simulink model "RRmanipulatorsim"  (R2020a)
settings: Solver=VariableStepAuto  StartTime=0.0  StopTime=7  RelTol=1e-3
values from neighbouring files (symbols this model uses):
  ike = ke^(-1)    (= 1e-06)    [RRmanipulator.m]    (also in RRmanipulator_.m)
  Ke = [1e6 0; 0 0]    [RRmanipulator.m]    (also in RRmanipulator_.m)
  ke = 1e6    (= 1000000)    [RRmanipulator.m]    (also in RRmanipulator_.m)
  Kp = [g1 0; 0 g2]    [RRmanipulator.m]    (also in RRmanipulator_.m)
  Kpf = [g1f 0; 0 g2f]    [RRmanipulator.m]    (also in RRmanipulator_.m)
  Kpf_ = g1f    (= 500000)    [RRmanipulator.m]    (also in RRmanipulator_.m)
  Kv = [2*sqrt(g1) 0; 0 2*sqrt(g2)]    [RRmanipulator.m]    (also in RRmanipulator_.m)
  Kvf = [2*sqrt(g1f) 0; 0 2*sqrt(g2f)]    [RRmanipulator.m]    (also in RRmanipulator_.m)
  R = [cos(-pi/4) -sin(-pi/4) ... (first row only)    [RRmanipulator.m]    (also in RRmanipulator_.m)
  RT = R'    [RRmanipulator.m]    (also in RRmanipulator_.m)
  S = [0 0; 0 1]    [RRmanipulator.m]    (also in RRmanipulator_.m)
  S_ = [1 0; 0 0]    [RRmanipulator.m]    (also in RRmanipulator_.m)
libraries: roblocks x29, simulink x11
(part 1 of 2)
settings Model: Creator=Tobias Scala  LastModifiedBy=Tobias Scala

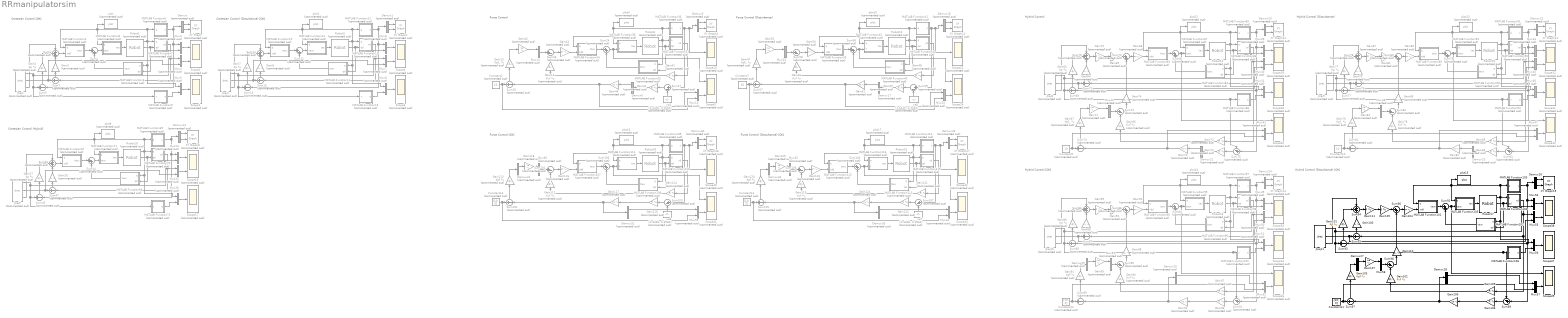
== system RRmanipulatorsim ==
  note: Cartesian Control [OK]
  note: Cartesian Control (Disturbance) [OK]
  note: Force Control
  note: Cartesian Control (Hybrid)
  note: Force Control (Disturbance)
  note: Hybrid Control
  note: Hybrid Control (Disturbance)
  note: Hybrid Control (Disturbance) [OK]
  note: Hybrid Control [OK]
  note: Force Control [OK]
  note: Force Control (Disturbance) [OK]
  Constant{2,7,9..10} (4 alike) : Constant  Commented=on  Value=10
  Constant11 : Constant  Value=[10; 0]
  Constant12 : Constant  Commented=on  Value=[10; 0]
  Constant13 : Constant  Commented=on  Value=[10; 0]
  Constant14 : Constant  Commented=on  Value=[10; 0]
  Demux{,1,5..6,13,16..17,20..25,29..35} (20 alike) : Demux  Commented=on  Outputs=2
  Demux26 : Demux  Outputs=2
  Demux27 : Demux  Outputs=2
  Demux28 : Demux  Outputs=2
  Gain100 : Gain  Gain=Kv  Multiplication=Matrix(K*u)
  Gain101 : Gain  Gain=Kp  Multiplication=Matrix(K*u)
  Gain102 : Gain  Gain=Kvf  Multiplication=Matrix(K*u)
  Gain103 : Gain  Gain=Kpf  Multiplication=Matrix(K*u)
  Gain104 : Gain  Gain=RT  Multiplication=Matrix(K*u)
  Gain105 : Gain  Gain=S  Multiplication=Matrix(K*u)
  Gain106 : Gain  Gain=Ke  Multiplication=Matrix(K*u)
  Gain107 : Gain  Gain=ike  Multiplication=Matrix(K*u)
  Gain108 : Gain  Gain=R  Multiplication=Matrix(K*u)
  Gain109 : Gain  Gain=R  Multiplication=Matrix(K*u)
  Gain110 : Gain  Gain=S_  Multiplication=Matrix(K*u)
  Gain111 : Gain  Gain=R  Multiplication=Matrix(K*u)
  Gain{12,46,66,78,90,112,119} (7 alike) : Gain  Commented=on  Gain=Kvf  Multiplication=Matrix(K*u)
  Gain113 : Gain  Commented=on  Gain=Kpf  Multiplication=Matrix(K*u)
  Gain{41..42,48..49,72..73,75,84..85,87,96..97,99,114..115,121..122} (17 alike) : Gain  Commented=on  Gain=R  Multiplication=Matrix(K*u)
  Gain{43,50,68,80,92,116,123} (7 alike) : Gain  Commented=on  Gain=RT  Multiplication=Matrix(K*u)
  Gain117 : Gain  Commented=on  Gain=Ke  Multiplication=Matrix(K*u)
  Gain{45,52,71,83,95,118,125} (7 alike) : Gain  Commented=on  Gain=ike  Multiplication=Matrix(K*u)
  Gain120 : Gain  Commented=on  Gain=Kpf  Multiplication=Matrix(K*u)
  Gain124 : Gain  Commented=on  Gain=Ke  Multiplication=Matrix(K*u)
  Gain{13,47,67,79} (4 alike) : Gain  Commented=on  Gain=Kpf_  Multiplication=Matrix(K*u)
  Gain{2,6,26,64,76,88} (6 alike) : Gain  Commented=on  Gain=Kv  Multiplication=Matrix(K*u)
  Gain{3,7,27,65,77,89} (6 alike) : Gain  Commented=on  Gain=Kp  Multiplication=Matrix(K*u)
  Gain{44,51,70,82} (4 alike) : Gain  Commented=on  Gain=ke  Multiplication=Matrix(K*u)
  Gain69 : Gain  Commented=on  Gain=S  Multiplication=Matrix(K*u)
  Gain74 : Gain  Commented=on  Gain=S_  Multiplication=Matrix(K*u)
  Gain81 : Gain  Commented=on  Gain=S  Multiplication=Matrix(K*u)
  Gain86 : Gain  Commented=on  Gain=S_  Multiplication=Matrix(K*u)
  Gain91 : Gain  Commented=on  Gain=Kpf  Multiplication=Matrix(K*u)
  Gain93 : Gain  Commented=on  Gain=S  Multiplication=Matrix(K*u)
  Gain94 : Gain  Commented=on  Gain=Ke  Multiplication=Matrix(K*u)
  Gain98 : Gain  Commented=on  Gain=S_  Multiplication=Matrix(K*u)
  MATLAB Function10 : MATLAB Function  Commented=on  TreatAsAtomicUnit=on
  MATLAB Function100 : MATLAB Function  Commented=on  TreatAsAtomicUnit=on
  MATLAB Function101 : MATLAB Function  TreatAsAtomicUnit=on
  MATLAB Function102 : MATLAB Function  TreatAsAtomicUnit=on
  MATLAB Function103 : MATLAB Function  TreatAsAtomicUnit=on
  MATLAB Function104 : MATLAB Function  TreatAsAtomicUnit=on
  MATLAB Function105 : MATLAB Function  TreatAsAtomicUnit=on
  MATLAB Function106 : MATLAB Function  TreatAsAtomicUnit=on
  MATLAB Function107 : MATLAB Function  Commented=on  TreatAsAtomicUnit=on
  MATLAB Function108 : MATLAB Function  Commented=on  TreatAsAtomicUnit=on
  MATLAB Function109 : MATLAB Function  Commented=on  TreatAsAtomicUnit=on
  MATLAB Function11 : MATLAB Function  Commented=on  TreatAsAtomicUnit=on
  MATLAB Function110 : MATLAB Function  Commented=on  TreatAsAtomicUnit=on
  MATLAB Function111 : MATLAB Function  Commented=on  TreatAsAtomicUnit=on
  MATLAB Function112 : MATLAB Function  Commented=on  TreatAsAtomicUnit=on
  MATLAB Function113 : MATLAB Function  Commented=on  TreatAsAtomicUnit=on
  MATLAB Function114 : MATLAB Function  Commented=on  TreatAsAtomicUnit=on
  MATLAB Function115 : MATLAB Function  Commented=on  TreatAsAtomicUnit=on
  MATLAB Function116 : MATLAB Function  Commented=on  TreatAsAtomicUnit=on
  MATLAB Function12 : MATLAB Function  Commented=on  TreatAsAtomicUnit=on
  MATLAB Function13 : MATLAB Function  Commented=on  TreatAsAtomicUnit=on
  MATLAB Function14 : MATLAB Function  Commented=on  TreatAsAtomicUnit=on
  MATLAB Function15 : MATLAB Function  Commented=on  TreatAsAtomicUnit=on
  MATLAB Function2 : MATLAB Function  Commented=on  TreatAsAtomicUnit=on
  MATLAB Function3 : MATLAB Function  Commented=on  TreatAsAtomicUnit=on
  MATLAB Function34 : MATLAB Function  Commented=on  TreatAsAtomicUnit=on
  MATLAB Function35 : MATLAB Function  Commented=on  TreatAsAtomicUnit=on
  MATLAB Function36 : MATLAB Function  Commented=on  TreatAsAtomicUnit=on
  MATLAB Function37 : MATLAB Function  Commented=on  TreatAsAtomicUnit=on
  MATLAB Function38 : MATLAB Function  Commented=on  TreatAsAtomicUnit=on
  MATLAB Function39 : MATLAB Function  Commented=on  TreatAsAtomicUnit=on
  MATLAB Function40 : MATLAB Function  Commented=on  TreatAsAtomicUnit=on
  MATLAB Function41 : MATLAB Function  Commented=on  TreatAsAtomicUnit=on
  MATLAB Function42 : MATLAB Function  Commented=on  TreatAsAtomicUnit=on
  MATLAB Function43 : MATLAB Function  Commented=on  TreatAsAtomicUnit=on
  MATLAB Function6 : MATLAB Function  Commented=on  TreatAsAtomicUnit=on
  MATLAB Function67 : MATLAB Function  Commented=on  TreatAsAtomicUnit=on
  MATLAB Function68 : MATLAB Function  Commented=on  TreatAsAtomicUnit=on
  MATLAB Function69 : MATLAB Function  Commented=on  TreatAsAtomicUnit=on
  MATLAB Function7 : MATLAB Function  Commented=on  TreatAsAtomicUnit=on
  MATLAB Function70 : MATLAB Function  Commented=on  TreatAsAtomicUnit=on
  MATLAB Function71 : MATLAB Function  Commented=on  TreatAsAtomicUnit=on
  MATLAB Function72 : MATLAB Function  Commented=on  TreatAsAtomicUnit=on
  MATLAB Function8 : MATLAB Function  Commented=on  TreatAsAtomicUnit=on
  MATLAB Function83 : MATLAB Function  Commented=on  TreatAsAtomicUnit=on
  MATLAB Function84 : MATLAB Function  Commented=on  TreatAsAtomicUnit=on
  MATLAB Function85 : MATLAB Function  Commented=on  TreatAsAtomicUnit=on
  MATLAB Function86 : MATLAB Function  Commented=on  TreatAsAtomicUnit=on
  MATLAB Function87 : MATLAB Function  Commented=on  TreatAsAtomicUnit=on
  MATLAB Function88 : MATLAB Function  Commented=on  TreatAsAtomicUnit=on
  MATLAB Function89 : MATLAB Function  Commented=on  TreatAsAtomicUnit=on
  MATLAB Function9 : MATLAB Function  Commented=on  TreatAsAtomicUnit=on
  MATLAB Function90 : MATLAB Function  Commented=on  TreatAsAtomicUnit=on
  MATLAB Function91 : MATLAB Function  Commented=on  TreatAsAtomicUnit=on
  MATLAB Function92 : MATLAB Function  Commented=on  TreatAsAtomicUnit=on
  MATLAB Function93 : MATLAB Function  Commented=on  TreatAsAtomicUnit=on
  MATLAB Function94 : MATLAB Function  Commented=on  TreatAsAtomicUnit=on
  MATLAB Function95 : MATLAB Function  Commented=on  TreatAsAtomicUnit=on
  MATLAB Function96 : MATLAB Function  Commented=on  TreatAsAtomicUnit=on
  MATLAB Function97 : MATLAB Function  Commented=on  TreatAsAtomicUnit=on
  MATLAB Function98 : MATLAB Function  Commented=on  TreatAsAtomicUnit=on
  MATLAB Function99 : MATLAB Function  Commented=on  TreatAsAtomicUnit=on
  Mux{3..8,13..14,24..26,32..33,39..53,59..62} (32 alike) : Mux  Commented=on  Inputs=2
  Mux{54..58} (5 alike) : Mux  Inputs=2
  Robot1 : roblocks/Arm/Robot  Commented=on  robot=RRbot  q0=[-pi/2 pi/2]
  Robot{6,10,14,16,18} (5 alike) : roblocks/Arm/Robot  Commented=on  robot=RRbot  q0=[-0.114*pi 0.364*pi]
  Robot12 : roblocks/Arm/Robot  Commented=on  robot=RRbotD  q0=[-0.114*pi 0.364*pi]
  Robot15 : roblocks/Arm/Robot  Commented=on  robot=RRbotD  q0=[-0.114*pi 0.364*pi]
  Robot17 : roblocks/Arm/Robot  robot=RRbotD  q0=[-0.114*pi 0.364*pi]
  Robot19 : roblocks/Arm/Robot  Commented=on  robot=RRbotD  q0=[-0.114*pi 0.364*pi]
  Robot3 : roblocks/Arm/Robot  Commented=on  robot=RRbotD  q0=[-pi/2 pi/2]
  Scope{1,3,10,17,23,28,31,34,40,42} (10 alike) : Scope  Commented=on
  Scope{2,4,9,19,24,29..30,32..33,35..36,41,43} (13 alike) : Scope  Commented=on  NumInputPorts=2
  Scope37 : Scope
  Scope38 : Scope  NumInputPorts=2
  Scope39 : Scope  NumInputPorts=2
  Sum{4,12,24,44,56,68,72,76,80,84,88,100,104} (13 alike) : Sum  Commented=on  Inputs=|++
  Sum{5,7,13,15,25,45,47,57,69,71,73,77,79,81,85,87,89,101,105} (19 alike) : Sum  Commented=on  Inputs=+|-
  Sum{26..27,58..59,74,82,90,102..103,106..107} (11 alike) : Sum  Commented=on  Inputs=|+-
  Sum{6,14,46,70,78,86} (6 alike) : Sum  Commented=on  Inputs=+++
  Sum75 : Sum  Commented=on  Inputs=-+|
  Sum83 : Sum  Commented=on  Inputs=-+|
  Sum91 : Sum  Commented=on  Inputs=-+|
  Sum92 : Sum  Inputs=|++
  Sum93 : Sum  Inputs=+|-
  Sum94 : Sum  Inputs=+++
  Sum95 : Sum  Inputs=+|-
  Sum96 : Sum  Inputs=|++
  Sum97 : Sum  Inputs=+|-
  Sum98 : Sum  Inputs=|+-
  Sum99 : Sum  Inputs=-+|
  XY Graph{,1,4,10,16..17} (6 alike) : simulink/Sinks/XY Graph  Commented=on  xmin=-1.5  xmax=1.5  ymin=-1.5  ymax=1.5  st=-1
  XY Graph{8,12..14} (4 alike) : simulink/Sinks/XY Graph  Commented=on  xmin=-2  xmax=2  ymin=-2  ymax=2  st=-1
  XY Graph15 : simulink/Sinks/XY Graph  xmin=-2  xmax=2  ymin=-2  ymax=2  st=-1
  jtraj1 : roblocks/Toolbox/jtraj  Commented=on  q0=[1 -1]  qf=[1 1]  tmax=2  ts=0.02
  jtraj{5,8..10} (4 alike) : roblocks/Toolbox/jtraj  Commented=on  q0=[1.6436 0.3564]  qf=[0.3564 1.6436]  tmax=2  ts=0.02
  jtraj11 : roblocks/Toolbox/jtraj  q0=[1.6436 0.3564]  qf=[0.3564 1.6436]  tmax=2  ts=0.02
  jtraj3 : roblocks/Toolbox/jtraj  Commented=on  q0=[1 -1]  qf=[1 1]  tmax=2  ts=0.02
  plot{,4,8,12,14,16} (6 alike) : roblocks/Arm/plot  Commented=on  robot=RRbot  fps=5  holdplot=on
  plot{1,10,13,17} (4 alike) : roblocks/Arm/plot  Commented=on  robot=RRbotD  fps=5  holdplot=on
  plot15 : roblocks/Arm/plot  robot=RRbotD  fps=5  holdplot=on
  xe{2,5..7} (4 alike) : Constant  Commented=on  Value=[1.6436; 0.3564]
  wires:
  jtraj1/3 -> Sum6/1
  jtraj1/1 -> MATLAB Function9/1(x), Sum5/1, Mux3/2
  Gain3/1 -> Sum6/2
  Sum7/1 -> Gain2/1
  jtraj1/2 -> Mux4/2, Sum7/1
  Sum5/1 -> Gain3/1
  Gain2/1 -> Sum6/3
  MATLAB Function3/1(taux) -> Sum4/2
  Robot1/1 -> MATLAB Function6/1(q), plot/1, MATLAB Function8/1(q), MATLAB Function2/1(q), Mux5/1, MATLAB Function3/1(q), MATLAB Function7/1(q)
  Robot1/2 -> MATLAB Function3/2(qd), MATLAB Function7/2(qd)
  Sum6/1 -> MATLAB Function2/2(xdd)
  MATLAB Function6/1(x) -> Demux/1, Sum5/2, Mux3/1
  MATLAB Function7/1(xd) -> Sum7/2, Mux4/1
  MATLAB Function2/1(taux) -> Sum4/1
  Sum4/1 -> MATLAB Function8/2(taux)
  MATLAB Function8/1(tau) -> Robot1/1
  Mux3/1 -> Scope2/1
  Mux4/1 -> Scope2/2
  Mux5/1 -> Scope1/1
  MATLAB Function9/1(q) -> Mux5/2
  Demux/2 -> XY Graph/2
  Demux/1 -> XY Graph/1
  MATLAB Function15/1(q) -> Mux8/2
  Demux1/2 -> XY Graph1/2
  MATLAB Function10/1(taux) -> Sum12/1
  Mux6/1 -> Scope4/1
  MATLAB Function14/1(tau) -> Robot3/1
  Mux8/1 -> Scope3/1
  Mux7/1 -> Scope4/2
  MATLAB Function12/1(x) -> Demux1/1, Sum13/2, Mux6/1
  Demux1/1 -> XY Graph1/1
  Robot3/2 -> MATLAB Function11/2(qd), MATLAB Function13/2(qd)
  Sum12/1 -> MATLAB Function14/2(taux)
  MATLAB Function13/1(xd) -> Sum15/2, Mux7/1
  Robot3/1 -> MATLAB Function12/1(q), plot1/1, MATLAB Function14/1(q), MATLAB Function10/1(q), Mux8/1, MATLAB Function11/1(q), MATLAB Function13/1(q)
  Sum14/1 -> MATLAB Function10/2(xdd)
  Sum13/1 -> Gain7/1
  Gain6/1 -> Sum14/3
  Gain7/1 -> Sum14/2
  jtraj3/3 -> Sum14/1
  jtraj3/2 -> Mux7/2, Sum15/1
  Sum15/1 -> Gain6/1
  jtraj3/1 -> MATLAB Function15/1(x), Sum13/1, Mux6/2
  MATLAB Function11/1(taux) -> Sum12/2
  MATLAB Function36/1(x) -> Demux5/1, Scope10/1, Sum27/1
  Constant2/1 -> Mux13/2, Sum25/1
  xe2/1 -> Sum27/2
  Sum27/1 -> Gain42/1
  Sum26/1 -> Gain43/1
  Gain44/1 -> Mux13/1, Sum25/2
  Gain45/1 -> Mux14/1
  Robot6/2 -> MATLAB Function35/2(qd), MATLAB Function37/2(qd)
  Sum24/1 -> Scope9/1, MATLAB Function38/2(f)
  Sum25/1 -> Gain13/1
  MATLAB Function34/1(taux) -> Sum24/1
  MATLAB Function35/1(taux) -> Sum24/2
  Demux6/1 -> Gain44/1
  MATLAB Function38/1(tau) -> Robot6/1
  Gain41/1 -> Gain12/1
  Demux5/1 -> XY Graph4/1
  Demux5/2 -> XY Graph4/2
  Gain43/1 -> MATLAB Function34/2(xdd)
  Gain12/1 -> Sum26/2
  MATLAB Function37/1(xd) -> Gain41/1
  Mux14/1 -> Sum26/1
  Robot6/1 -> MATLAB Function36/1(q), MATLAB Function38/1(q), MATLAB Function34/1(q), plot4/1, MATLAB Function35/1(q), MATLAB Function37/1(q)
  Gain42/1 -> Demux6/1
  Gain13/1 -> Gain45/1
  Mux13/1 -> Scope9/2
  Robot10/2 -> MATLAB Function68/2(qd), MATLAB Function70/2(qd)
  MATLAB Function67/1(taux) -> Sum44/1
  Sum44/1 -> MATLAB Function71/2(taux)
  Mux25/1 -> Scope19/2
  Sum46/1 -> MATLAB Function67/2(xdd)
  Gain27/1 -> Sum46/2
  Sum45/1 -> Gain27/1
  MATLAB Function70/1(xd) -> Sum47/2, Mux25/1
  MATLAB Function71/1(tau) -> Robot10/1
  MATLAB Function69/1(x) -> Demux13/1, Sum45/2, Mux24/1
  Robot10/1 -> MATLAB Function69/1(q), plot8/1, MATLAB Function71/1(q), MATLAB Function67/1(q), Mux26/1, MATLAB Function68/1(q), MATLAB Function70/1(q)
  Mux24/1 -> Scope19/1
  Mux26/1 -> Scope17/1
  Gain26/1 -> Sum46/3
  jtraj5/2 -> Mux25/2, Sum47/1
  Demux13/2 -> XY Graph8/2
  Sum47/1 -> Gain26/1
  MATLAB Function68/1(taux) -> Sum44/2
  Demux13/1 -> XY Graph8/1
  jtraj5/1 -> MATLAB Function72/1(x), Sum45/1, Mux24/2
  MATLAB Function72/1(q) -> Mux26/2
  jtraj5/3 -> Sum46/1
  Gain51/1 -> Mux32/1, Sum57/2
  Demux17/1 -> Gain51/1
  Gain49/1 -> Demux17/1
  MATLAB Function42/1(xd) -> Gain48/1
  Gain52/1 -> Mux33/1
  Gain47/1 -> Gain52/1
  Demux16/2 -> XY Graph10/2
  Sum56/1 -> Scope24/1, MATLAB Function43/2(f)
  Sum58/1 -> Gain50/1
  Mux33/1 -> Sum58/1
  Gain48/1 -> Gain46/1
  Mux32/1 -> Scope24/2
  Robot12/1 -> MATLAB Function41/1(q), MATLAB Function43/1(q), MATLAB Function39/1(q), plot10/1, MATLAB Function40/1(q), MATLAB Function42/1(q)
  Gain46/1 -> Sum58/2
  Demux16/1 -> XY Graph10/1
  MATLAB Function43/1(tau) -> Robot12/1
  Constant7/1 -> Mux32/2, Sum57/1
  MATLAB Function39/1(taux) -> Sum56/1
  xe5/1 -> Sum59/2
  Sum59/1 -> Gain49/1
  MATLAB Function41/1(x) -> Demux16/1, Scope23/1, Sum59/1
  Robot12/2 -> MATLAB Function40/2(qd), MATLAB Function42/2(qd)
  Gain50/1 -> MATLAB Function39/2(xdd)
  Sum57/1 -> Gain47/1
  MATLAB Function40/1(taux) -> Sum56/2
  Gain73/1 -> Gain66/1
  Gain66/1 -> Sum74/2
  MATLAB Function88/1(q) -> Mux41/2
  MATLAB Function87/1(tau) -> Robot14/1
  Demux21/1 -> Gain70/1
  MATLAB Function84/1(taux) -> Sum68/2
  Mux43/1 -> Sum74/1
  Gain70/1 -> Mux42/1, Sum73/2
  Sum75/1 -> Gain72/1
  Mux42/1 -> Scope30/2
  Sum71/1 -> Gain64/1
  Gain65/1 -> Sum70/2
  Robot14/1 -> MATLAB Function85/1(q), plot12/1, MATLAB Function87/1(q), MATLAB Function83/1(q), Mux41/1, MATLAB Function84/1(q), MATLAB Function86/1(q)
  Gain72/1 -> Demux21/1
  MATLAB Function85/1(x) -> Sum75/2, Sum69/2, Mux39/1, Demux20/1
  Constant9/1 -> Mux42/2, Sum73/1
  Demux20/2 -> XY Graph12/2
  Mux41/1 -> Scope28/1
  Gain64/1 -> Sum70/3
  Gain71/1 -> Mux43/1
  Sum68/1 -> Scope30/1, MATLAB Function87/2(taux)
  MATLAB Function83/1(taux) -> Sum68/1
  Sum74/1 -> Gain74/1
  Gain74/1 -> Sum72/2
  Sum69/1 -> Gain65/1
  Sum73/1 -> Gain67/1
  Gain69/1 -> Sum72/1
  MATLAB Function86/1(xd) -> Sum71/2, Gain73/1, Mux40/1
  Gain67/1 -> Gain71/1
  Demux20/1 -> XY Graph12/1
  Sum72/1 -> Gain68/1
  Sum70/1 -> Gain75/1
  Mux40/1 -> Scope29/2
  Robot14/2 -> MATLAB Function84/2(qd), MATLAB Function86/2(qd)
  Mux39/1 -> Scope29/1
  jtraj8/1 -> Mux39/2, Sum69/1, MATLAB Function88/1(x), Sum75/1
  jtraj8/2 -> Mux40/2, Sum71/1
  jtraj8/3 -> Sum70/1
  Gain68/1 -> MATLAB Function83/2(xdd)
  Gain75/1 -> Gain69/1
  Gain87/1 -> Gain81/1
  Mux45/1 -> Scope32/2
  Sum78/1 -> Gain87/1
  Sum80/1 -> Gain80/1
  Demux22/1 -> XY Graph13/1
  Gain79/1 -> Gain83/1
  MATLAB Function92/1(xd) -> Sum79/2, Gain85/1, Mux45/1
  MATLAB Function89/1(taux) -> Sum76/1
  Gain83/1 -> Mux48/1
  Sum76/1 -> Scope33/1, MATLAB Function93/2(taux)
  Demux22/2 -> XY Graph13/2
  Constant10/1 -> Mux47/2, Sum81/1
  Gain76/1 -> Sum78/3
  Sum82/1 -> Gain86/1
  Sum81/1 -> Gain79/1
  Gain77/1 -> Sum78/2
  Sum79/1 -> Gain76/1
  Mux47/1 -> Scope33/2
  Gain82/1 -> Mux47/1, Sum81/2
  Gain84/1 -> Demux23/1
  Gain81/1 -> Sum80/1
  MATLAB Function90/1(taux) -> Sum76/2
  Robot15/1 -> MATLAB Function91/1(q), plot13/1, MATLAB Function93/1(q), MATLAB Function89/1(q), Mux46/1, MATLAB Function90/1(q), MATLAB Function92/1(q)
  Sum77/1 -> Gain77/1
  Sum83/1 -> Gain84/1
  MATLAB Function93/1(tau) -> Robot15/1
  Demux23/1 -> Gain82/1
  Gain78/1 -> Sum82/2
  Gain85/1 -> Gain78/1
  MATLAB Function94/1(q) -> Mux46/2
  Robot15/2 -> MATLAB Function90/2(qd), MATLAB Function92/2(qd)
  jtraj9/2 -> Mux45/2, Sum79/1
  Mux48/1 -> Sum82/1
  jtraj9/1 -> Mux44/2, Sum77/1, MATLAB Function94/1(x), Sum83/1
  Mux46/1 -> Scope31/1
  jtraj9/3 -> Sum78/1
  Gain86/1 -> Sum80/2
  Mux44/1 -> Scope32/1
  Gain80/1 -> MATLAB Function89/2(xdd)
  MATLAB Function91/1(x) -> Sum83/2, Sum77/2, Mux44/1, Demux22/1
  Gain105/1 -> Sum96/1
  MATLAB Function102/1(taux) -> Sum92/2
  Sum98/1 -> Gain110/1
  Gain101/1 -> Sum94/2
  Sum97/1 -> Gain103/1
  Gain106/1 -> Demux28/1, Sum97/2
  Mux57/1 -> Scope39/2
  Sum95/1 -> Gain100/1
  Gain100/1 -> Sum94/3
  Demux26/2 -> XY Graph15/2
  Sum92/1 -> Scope39/1, MATLAB Function105/2(taux)
  MATLAB Function104/1(xd) -> Sum95/2, Gain109/1, Mux55/1
  MATLAB Function101/1(taux) -> Sum92/1
  Gain107/1 -> Mux58/1
  Sum99/1 -> Gain108/1
  Sum93/1 -> Gain101/1
  Robot17/1 -> MATLAB Function103/1(q), plot15/1, MATLAB Function105/1(q), MATLAB Function101/1(q), Mux56/1, MATLAB Function102/1(q), MATLAB Function104/1(q)
  Mux55/1 -> Scope38/2
  Constant11/1 -> Mux57/2, Sum97/1
  Sum94/1 -> Gain111/1
  Gain109/1 -> Gain102/1
  Gain102/1 -> Sum98/2
  jtraj11/2 -> Mux55/2, Sum95/1
  Robot17/2 -> MATLAB Function102/2(qd), MATLAB Function104/2(qd)
  Gain111/1 -> Gain105/1
  Gain110/1 -> Sum96/2
  Mux56/1 -> Scope37/1
  jtraj11/3 -> Sum94/1
  jtraj11/1 -> Mux54/2, Sum93/1, MATLAB Function106/1(x), Sum99/1
  Gain104/1 -> MATLAB Function101/2(xdd)
  MATLAB Function106/1(q) -> Mux56/2
  Mux58/1 -> Sum98/1
  MATLAB Function103/1(x) -> Sum99/2, Sum93/2, Mux54/1, Demux26/1
  Demux26/1 -> XY Graph15/1
  Sum96/1 -> Gain104/1
  Gain108/1 -> Gain106/1
  MATLAB Function105/1(tau) -> Robot17/1
  Mux54/1 -> Scope38/1
  Demux27/1 -> Gain107/1
  Gain103/1 -> Demux27/1
  Demux28/1 -> Mux57/1
  Mux49/1 -> Scope35/1
  Sum88/1 -> Gain92/1
  Demux24/1 -> XY Graph14/1
  MATLAB Function97/1(x) -> Sum91/2, Sum85/2, Mux49/1, Demux24/1
  Mux53/1 -> Sum90/1
  jtraj10/1 -> Mux49/2, Sum85/1, MATLAB Function100/1(x), Sum91/1
  Gain96/1 -> Gain94/1
  Gain99/1 -> Gain93/1
  Gain90/1 -> Sum90/2
  Gain97/1 -> Gain90/1
  MATLAB Function100/1(q) -> Mux51/2
  Mux50/1 -> Scope35/2
  Robot16/1 -> MATLAB Function97/1(q), plot14/1, MATLAB Function99/1(q), MATLAB Function95/1(q), Mux51/1, MATLAB Function96/1(q), MATLAB Function98/1(q)
  Gain92/1 -> MATLAB Function95/2(xdd)
  Sum85/1 -> Gain89/1
  jtraj10/2 -> Mux50/2, Sum87/1
  Robot16/2 -> MATLAB Function96/2(qd), MATLAB Function98/2(qd)
  Sum91/1 -> Gain96/1
  Gain95/1 -> Mux53/1
  jtraj10/3 -> Sum86/1
  Gain98/1 -> Sum88/2
  Constant12/1 -> Mux52/2, Sum89/1
  Mux51/1 -> Scope34/1
  Gain91/1 -> Demux25/1
  Demux29/1 -> Mux52/1
  MATLAB Function95/1(taux) -> Sum84/1
  Sum86/1 -> Gain99/1
  MATLAB Function99/1(tau) -> Robot16/1
  Sum84/1 -> Scope36/1, MATLAB Function99/2(taux)
  Demux24/2 -> XY Graph14/2
  Gain88/1 -> Sum86/3
  MATLAB Function98/1(xd) -> Sum87/2, Gain97/1, Mux50/1
  Sum87/1 -> Gain88/1
  Mux52/1 -> Scope36/2
  Gain89/1 -> Sum86/2
  Sum89/1 -> Gain91/1
  Sum90/1 -> Gain98/1
  MATLAB Function96/1(taux) -> Sum84/2
  Gain94/1 -> Demux29/1, Sum89/2
  Demux25/1 -> Gain95/1
  Gain93/1 -> Sum88/1
  Sum100/1 -> Scope41/1, MATLAB Function111/2(f)
  Gain114/1 -> Gain112/1
  Sum103/1 -> Gain115/1
  Robot18/1 -> MATLAB Function109/1(q), MATLAB Function111/1(q), MATLAB Function107/1(q), plot16/1, MATLAB Function108/1(q), MATLAB Function110/1(q)
  Sum102/1 -> Gain116/1
  Gain118/1 -> Mux60/1
  MATLAB Function109/1(x) -> Demux30/1, Scope40/1, Sum103/1
  Sum101/1 -> Gain113/1
  Constant13/1 -> Mux59/2, Sum101/1
  MATLAB Function111/1(tau) -> Robot18/1
  Robot18/2 -> MATLAB Function108/2(qd), MATLAB Function110/2(qd)
  Gain116/1 -> MATLAB Function107/2(xdd)
  MATLAB Function107/1(taux) -> Sum100/1
  MATLAB Function108/1(taux) -> Sum100/2
  Mux60/1 -> Sum102/1
  Gain117/1 -> Demux32/1, Sum101/2
  Mux59/1 -> Scope41/2
  MATLAB Function110/1(xd) -> Gain114/1
  Demux30/1 -> XY Graph16/1
  Gain115/1 -> Gain117/1
  xe6/1 -> Sum103/2
  Gain112/1 -> Sum102/2
  Demux30/2 -> XY Graph16/2
  Demux31/1 -> Gain118/1
  Gain113/1 -> Demux31/1
  Demux32/1 -> Mux59/1
  Demux33/2 -> XY Graph17/2
  MATLAB Function113/1(taux) -> Sum104/2
  Gain124/1 -> Demux35/1, Sum105/2
  Gain123/1 -> MATLAB Function112/2(xdd)
  Robot19/2 -> MATLAB Function113/2(qd), MATLAB Function115/2(qd)
  Mux61/1 -> Scope43/2
  xe7/1 -> Sum107/2
  MATLAB Function114/1(x) -> Demux33/1, Scope42/1, Sum107/1
  MATLAB Function116/1(tau) -> Robot19/1
  Gain125/1 -> Mux62/1
  Sum105/1 -> Gain120/1
  Sum106/1 -> Gain123/1
  Demux33/1 -> XY Graph17/1
  Robot19/1 -> MATLAB Function114/1(q), MATLAB Function116/1(q), MATLAB Function112/1(q), plot17/1, MATLAB Function113/1(q), MATLAB Function115/1(q)
  Gain119/1 -> Sum106/2
  MATLAB Function115/1(xd) -> Gain121/1
  Constant14/1 -> Mux61/2, Sum105/1
  Sum104/1 -> Scope43/1, MATLAB Function116/2(f)
  Mux62/1 -> Sum106/1
  Gain120/1 -> Demux34/1
  MATLAB Function112/1(taux) -> Sum104/1
  Sum107/1 -> Gain122/1
  Demux35/1 -> Mux61/1
  Gain121/1 -> Gain119/1
  Demux34/1 -> Gain125/1
  Gain122/1 -> Gain124/1

== matlab function RRmanipulatorsim/MATLAB Function34 ==
  data: q input; taux output; xdd input
function taux = Mx(q, xdd)
    L = [1 1]; %Links long.
    m = [1 1]; %Links weight.
    
    M = [L(2)*m(2)*(L(2)+cos(q(2))*L(1))+m(1)*L(1)^2+L(1)*m(2)*(L(1)+cos(q(2))*L(2)) L(2)^2*m(2)+L(1)*m(2)*L(2)*cos(q(2));
        L(2)*m(2)*(L(2)+cos(q(2))*L(1)) L(2)^2*m(2)];
    J = [-sin(sum(q))*L(2)-sin(q(1))*L(1) -sin(sum(q))*L(2);
        cos(sum(q))*L(2)+cos(q(1))*L(1) cos(sum(q))*L(2)];
    iJ = J^(-1);
    iJT = (J.')^(-1);
    
    Mx = iJT*M*iJ;
taux = [Mx(1,1)*xdd(1)+Mx(1,2)*xdd(2); Mx(2,1)*xdd(1)+Mx(2,2)*xdd(2)];

% function taux = Mx(q, xdd)
%     M = RRbot.inertia(q');
%     J = RRbot.jacob0(q');
%     J = J(1:N,1:N);
%     iJ = J^(-1);
%     iJT = J.'^(-1);
%     
%     Mx = iJT*M.*iJ;
% taux = [Mx(1,1)*xdd(1)+Mx(1,2)*xdd(2); Mx(2,1)*xdd(1)+Mx(2,2)*xdd(2)];

== matlab function RRmanipulatorsim/MATLAB Function35 ==
  data: q input; taux output; qd input
function taux = Vx_Fx(q, qd)
    L = [1 1]; %Links long.
    m = [1 1]; %Links weight.
    
    M = [L(2)*m(2)*(L(2)+cos(q(2))*L(1))+m(1)*L(1)^2+L(1)*m(2)*(L(1)+cos(q(2))*L(2)) L(2)^2*m(2)+L(1)*m(2)*L(2)*cos(q(2));
        L(2)*m(2)*(L(2)+cos(q(2))*L(1)) L(2)^2*m(2)];
    V = [-2*m(2)*L(1)*L(2)*sin(q(2))*prod(qd)-m(2)*L(1)*L(2)*sin(q(2))*qd(2)^2;
        m(2)*L(1)*L(2)*sin(q(2))*qd(1)^2];
    G = [0;
        0];
    F = [sign(qd(1));
        sign(qd(2))];
    J = [-sin(sum(q))*L(2)-sin(q(1))*L(1) -sin(sum(q))*L(2);
        cos(sum(q))*L(2)+cos(q(1))*L(1) cos(sum(q))*L(2)];
    iJ = J^(-1);
    iJT = (J')^(-1);
    dJ = [-(sum(qd))*cos(sum(q))*L(2)-qd(1)*cos(q(1))*L(1) -(sum(qd))*cos(sum(q))*L(2);
        -(sum(qd))*sin(sum(q))*L(2)-qd(1)*sin(q(1))*L(1) -(sum(qd))*sin(sum(q))*L(2)];
    
    %dJqd = [dJ(1,1)*qd(1)+dJ(1,2)*qd(2); dJ(2,1)*qd(1)+dJ(2,2)*qd(2)];
    Vx = M*iJ*dJ;
    Vx = V - [Vx(1,1)*qd(1)+Vx(1,2)*qd(2); Vx(2,1)*qd(1)+Vx(2,2)*qd(2)];
    Vx = [iJT(1,1)*Vx(1)+iJT(1,2)*Vx(2); iJT(2,1)*Vx(1)+iJT(2,2)*Vx(2)];
    Gx = [iJT(1,1)*G(1)+iJT(1,2)*G(2); iJT(2,1)*G(1)+iJT(2,2)*G(2)];
    Fx = [iJT(1,1)*F(1)+iJT(1,2)*F(2); iJT(2,1)*F(1)+iJT(2,2)*F(2)];
taux = Vx + Gx + Fx;

% function taux = Vx_Fx(q, qd)
%     C = RRbot.coriolis(q', qd');
%     V = [C(1,1)*qd(1)+C(1,2)*qd(2); C(2,1)*qd(1)+C(2,2)*qd(2)]; %V = Cqd
%     F = -RRbot.friction(qd')';
%     J = RRbot.jacob0(q');
%     J = J(1:N,1:N);
%     iJ = J^(-1);
%     iJT = J.'^(-1);
%     dJ = [-(sum(qd))*cos(sum(q))*LT-qd(1)*cos(q(1))*L1 -(sum(qd))*cos(sum(q))*LT;
%         -(sum(qd))*sin(sum(q))*LT-qd(1)*sin(q(1))*L1 -(sum(qd))*sin(sum(q))*LT];
%     dJqd = [dJ(1,1)*qd(1)+dJ(1,2)*qd(2); dJ(2,1)*qd(1)+dJ(2,2)*qd(2)];
%     
%     Vx = M*iJ;
%     Vx = V - [Vx(1,1)*dJqd(1)+Vx(1,2)*dJqd(2); Vx(2,1)*dJqd(1)+Vx(2,2)*dJqd(2)];
%     Vx = [iJT(1,1)*Vx(1)+iJT(1,2)*Vx(2); iJT(2,1)*Vx(1)+iJT(2,2)*Vx(2)];
%     Fx = [iJT(1,1)*F(1)+iJT(1,2)*F(2); iJT(2,1)*F(1)+iJT(2,2)*F(2)];
% taux = Vx + Fx;

== matlab function RRmanipulatorsim/MATLAB Function36 ==
  data: q input; x output
function x = kine(q)
    L = [1 1]; %Links long.

x = [cos(sum(q))*L(2)+cos(q(1))*L(1); sin(sum(q))*L(2)+sin(q(1))*L(1)];

== matlab function RRmanipulatorsim/MATLAB Function37 ==
  data: q input; xd output; qd input
function xd = J(q, qd)
    L = [1 1]; %Links long.

    J = [-sin(sum(q))*L(2)-sin(q(1))*L(1) -sin(sum(q))*L(2);
        cos(sum(q))*L(2)+cos(q(1))*L(1) cos(sum(q))*L(2)];
xd = [J(1,1)*qd(1)+J(1,2)*qd(2); J(2,1)*qd(1)+J(2,2)*qd(2)];

== matlab function RRmanipulatorsim/MATLAB Function38 ==
  data: q input; tau output; f input
function tau = JT(q, f)    
    L = [1 1]; %Links long.

    J = [-sin(sum(q))*L(2)-sin(q(1))*L(1) -sin(sum(q))*L(2);
        cos(sum(q))*L(2)+cos(q(1))*L(1) cos(sum(q))*L(2)];
    JT = J';
tau = [JT(1,1)*f(1)+JT(1,2)*f(2); JT(2,1)*f(1)+JT(2,2)*f(2)];

% function tau = JT(q, taux)
%     J = RRbot.jacob0(q');
%     JT = J(1:N,1:N)';
% tau = [JT(1,1)*taux(1)+JT(1,2)*taux(2); JT(2,1)*taux(1)+JT(2,2)*taux(2)];

== matlab function RRmanipulatorsim/MATLAB Function39 ==
  data: q input; taux output; xdd input
function taux = Mx(q, xdd)
    L = [1 1]; %Links long.
    m = [1 1]; %Links weight.
    
    M = [L(2)*m(2)*(L(2)+cos(q(2))*L(1))+m(1)*L(1)^2+L(1)*m(2)*(L(1)+cos(q(2))*L(2)) L(2)^2*m(2)+L(1)*m(2)*L(2)*cos(q(2));
        L(2)*m(2)*(L(2)+cos(q(2))*L(1)) L(2)^2*m(2)];
    J = [-sin(sum(q))*L(2)-sin(q(1))*L(1) -sin(sum(q))*L(2);
        cos(sum(q))*L(2)+cos(q(1))*L(1) cos(sum(q))*L(2)];
    iJ = J^(-1);
    iJT = (J.')^(-1);
    
    Mx = iJT*M*iJ;
taux = [Mx(1,1)*xdd(1)+Mx(1,2)*xdd(2); Mx(2,1)*xdd(1)+Mx(2,2)*xdd(2)];

% function taux = Mx(q, xdd)
%     M = RRbot.inertia(q');
%     J = RRbot.jacob0(q');
%     J = J(1:N,1:N);
%     iJ = J^(-1);
%     iJT = J.'^(-1);
%     
%     Mx = iJT*M.*iJ;
% taux = [Mx(1,1)*xdd(1)+Mx(1,2)*xdd(2); Mx(2,1)*xdd(1)+Mx(2,2)*xdd(2)];

== matlab function RRmanipulatorsim/MATLAB Function40 ==
  data: q input; taux output; qd input
function taux = Vx_Fx(q, qd)
    L = [1 1]; %Links long.
    m = [1 1]; %Links weight.
    
    M = [L(2)*m(2)*(L(2)+cos(q(2))*L(1))+m(1)*L(1)^2+L(1)*m(2)*(L(1)+cos(q(2))*L(2)) L(2)^2*m(2)+L(1)*m(2)*L(2)*cos(q(2));
        L(2)*m(2)*(L(2)+cos(q(2))*L(1)) L(2)^2*m(2)];
    V = [-2*m(2)*L(1)*L(2)*sin(q(2))*prod(qd)-m(2)*L(1)*L(2)*sin(q(2))*qd(2)^2;
        m(2)*L(1)*L(2)*sin(q(2))*qd(1)^2];
    G = [0;
        0];
    F = [sign(qd(1));
        sign(qd(2))];
    J = [-sin(sum(q))*L(2)-sin(q(1))*L(1) -sin(sum(q))*L(2);
        cos(sum(q))*L(2)+cos(q(1))*L(1) cos(sum(q))*L(2)];
    iJ = J^(-1);
    iJT = (J')^(-1);
    dJ = [-(sum(qd))*cos(sum(q))*L(2)-qd(1)*cos(q(1))*L(1) -(sum(qd))*cos(sum(q))*L(2);
        -(sum(qd))*sin(sum(q))*L(2)-qd(1)*sin(q(1))*L(1) -(sum(qd))*sin(sum(q))*L(2)];
    
    %dJqd = [dJ(1,1)*qd(1)+dJ(1,2)*qd(2); dJ(2,1)*qd(1)+dJ(2,2)*qd(2)];
    Vx = M*iJ*dJ;
    Vx = V - [Vx(1,1)*qd(1)+Vx(1,2)*qd(2); Vx(2,1)*qd(1)+Vx(2,2)*qd(2)];
    Vx = [iJT(1,1)*Vx(1)+iJT(1,2)*Vx(2); iJT(2,1)*Vx(1)+iJT(2,2)*Vx(2)];
    Gx = [iJT(1,1)*G(1)+iJT(1,2)*G(2); iJT(2,1)*G(1)+iJT(2,2)*G(2)];
    Fx = [iJT(1,1)*F(1)+iJT(1,2)*F(2); iJT(2,1)*F(1)+iJT(2,2)*F(2)];
taux = Vx + Gx + Fx;

% function taux = Vx_Fx(q, qd)
%     C = RRbot.coriolis(q', qd');
%     V = [C(1,1)*qd(1)+C(1,2)*qd(2); C(2,1)*qd(1)+C(2,2)*qd(2)]; %V = Cqd
%     F = -RRbot.friction(qd')';
%     J = RRbot.jacob0(q');
%     J = J(1:N,1:N);
%     iJ = J^(-1);
%     iJT = J.'^(-1);
%     dJ = [-(sum(qd))*cos(sum(q))*LT-qd(1)*cos(q(1))*L1 -(sum(qd))*cos(sum(q))*LT;
%         -(sum(qd))*sin(sum(q))*LT-qd(1)*sin(q(1))*L1 -(sum(qd))*sin(sum(q))*LT];
%     dJqd = [dJ(1,1)*qd(1)+dJ(1,2)*qd(2); dJ(2,1)*qd(1)+dJ(2,2)*qd(2)];
%     
%     Vx = M*iJ;
%     Vx = V - [Vx(1,1)*dJqd(1)+Vx(1,2)*dJqd(2); Vx(2,1)*dJqd(1)+Vx(2,2)*dJqd(2)];
%     Vx = [iJT(1,1)*Vx(1)+iJT(1,2)*Vx(2); iJT(2,1)*Vx(1)+iJT(2,2)*Vx(2)];
%     Fx = [iJT(1,1)*F(1)+iJT(1,2)*F(2); iJT(2,1)*F(1)+iJT(2,2)*F(2)];
% taux = Vx + Fx;

== matlab function RRmanipulatorsim/MATLAB Function41 ==
  data: q input; x output
function x = kine(q)
    L = [1 1]; %Links long.

x = [cos(sum(q))*L(2)+cos(q(1))*L(1); sin(sum(q))*L(2)+sin(q(1))*L(1)];

== matlab function RRmanipulatorsim/MATLAB Function42 ==
  data: q input; xd output; qd input
function xd = J(q, qd)
    L = [1 1]; %Links long.

    J = [-sin(sum(q))*L(2)-sin(q(1))*L(1) -sin(sum(q))*L(2);
        cos(sum(q))*L(2)+cos(q(1))*L(1) cos(sum(q))*L(2)];
xd = [J(1,1)*qd(1)+J(1,2)*qd(2); J(2,1)*qd(1)+J(2,2)*qd(2)];

== matlab function RRmanipulatorsim/MATLAB Function3 ==
  data: q input; taux output; qd input
function taux = Vx_Fx(q, qd)
    L = [1 1]; %Links long.
    m = [1 1]; %Links weight.
    
    M = [L(2)*m(2)*(L(2)+cos(q(2))*L(1))+m(1)*L(1)^2+L(1)*m(2)*(L(1)+cos(q(2))*L(2)) L(2)^2*m(2)+L(1)*m(2)*L(2)*cos(q(2));
        L(2)*m(2)*(L(2)+cos(q(2))*L(1)) L(2)^2*m(2)];
    V = [-2*m(2)*L(1)*L(2)*sin(q(2))*prod(qd)-m(2)*L(1)*L(2)*sin(q(2))*qd(2)^2;
        m(2)*L(1)*L(2)*sin(q(2))*qd(1)^2];
    G = [0;
        0];
    F = [sign(qd(1));
        sign(qd(2))];
    J = [-sin(sum(q))*L(2)-sin(q(1))*L(1) -sin(sum(q))*L(2);
        cos(sum(q))*L(2)+cos(q(1))*L(1) cos(sum(q))*L(2)];
    iJ = J^(-1);
    iJT = (J')^(-1);
    dJ = [-(sum(qd))*cos(sum(q))*L(2)-qd(1)*cos(q(1))*L(1) -(sum(qd))*cos(sum(q))*L(2);
        -(sum(qd))*sin(sum(q))*L(2)-qd(1)*sin(q(1))*L(1) -(sum(qd))*sin(sum(q))*L(2)];
    
    %dJqd = [dJ(1,1)*qd(1)+dJ(1,2)*qd(2); dJ(2,1)*qd(1)+dJ(2,2)*qd(2)];
    Vx = M*iJ*dJ;
    Vx = V - [Vx(1,1)*qd(1)+Vx(1,2)*qd(2); Vx(2,1)*qd(1)+Vx(2,2)*qd(2)];
    Vx = [iJT(1,1)*Vx(1)+iJT(1,2)*Vx(2); iJT(2,1)*Vx(1)+iJT(2,2)*Vx(2)];
    Gx = [iJT(1,1)*G(1)+iJT(1,2)*G(2); iJT(2,1)*G(1)+iJT(2,2)*G(2)];
    Fx = [iJT(1,1)*F(1)+iJT(1,2)*F(2); iJT(2,1)*F(1)+iJT(2,2)*F(2)];
taux = Vx + Gx + Fx;

% function taux = Vx_Fx(q, qd)
%     C = RRbot.coriolis(q', qd');
%     V = [C(1,1)*qd(1)+C(1,2)*qd(2); C(2,1)*qd(1)+C(2,2)*qd(2)]; %V = Cqd
%     F = -RRbot.friction(qd')';
%     J = RRbot.jacob0(q');
%     J = J(1:N,1:N);
%     iJ = J^(-1);
%     iJT = J.'^(-1);
%     dJ = [-(sum(qd))*cos(sum(q))*LT-qd(1)*cos(q(1))*L1 -(sum(qd))*cos(sum(q))*LT;
%         -(sum(qd))*sin(sum(q))*LT-qd(1)*sin(q(1))*L1 -(sum(qd))*sin(sum(q))*LT];
%     dJqd = [dJ(1,1)*qd(1)+dJ(1,2)*qd(2); dJ(2,1)*qd(1)+dJ(2,2)*qd(2)];
%     
%     Vx = M*iJ;
%     Vx = V - [Vx(1,1)*dJqd(1)+Vx(1,2)*dJqd(2); Vx(2,1)*dJqd(1)+Vx(2,2)*dJqd(2)];
%     Vx = [iJT(1,1)*Vx(1)+iJT(1,2)*Vx(2); iJT(2,1)*Vx(1)+iJT(2,2)*Vx(2)];
%     Fx = [iJT(1,1)*F(1)+iJT(1,2)*F(2); iJT(2,1)*F(1)+iJT(2,2)*F(2)];
% taux = Vx + Fx;

== matlab function RRmanipulatorsim/MATLAB Function43 ==
  data: q input; tau output; f input
function tau = JT(q, f)    
    L = [1 1]; %Links long.

    J = [-sin(sum(q))*L(2)-sin(q(1))*L(1) -sin(sum(q))*L(2);
        cos(sum(q))*L(2)+cos(q(1))*L(1) cos(sum(q))*L(2)];
    JT = J';
tau = [JT(1,1)*f(1)+JT(1,2)*f(2); JT(2,1)*f(1)+JT(2,2)*f(2)];

% function tau = JT(q, taux)
%     J = RRbot.jacob0(q');
%     JT = J(1:N,1:N)';
% tau = [JT(1,1)*taux(1)+JT(1,2)*taux(2); JT(2,1)*taux(1)+JT(2,2)*taux(2)];

== matlab function RRmanipulatorsim/MATLAB Function67 ==
  data: q input; taux output; xdd input
function taux = Mx(q, xdd)
    L = [1 1]; %Links long.
    m = [1 1]; %Links weight.
    
    M = [L(2)*m(2)*(L(2)+cos(q(2))*L(1))+m(1)*L(1)^2+L(1)*m(2)*(L(1)+cos(q(2))*L(2)) L(2)^2*m(2)+L(1)*m(2)*L(2)*cos(q(2));
        L(2)*m(2)*(L(2)+cos(q(2))*L(1)) L(2)^2*m(2)];
    J = [-sin(sum(q))*L(2)-sin(q(1))*L(1) -sin(sum(q))*L(2);
        cos(sum(q))*L(2)+cos(q(1))*L(1) cos(sum(q))*L(2)];
    iJ = J^(-1);
    iJT = (J.')^(-1);
    
    Mx = iJT*M*iJ;
taux = [Mx(1,1)*xdd(1)+Mx(1,2)*xdd(2); Mx(2,1)*xdd(1)+Mx(2,2)*xdd(2)];

% function taux = Mx(q, xdd)
%     M = RRbot.inertia(q');
%     J = RRbot.jacob0(q');
%     J = J(1:N,1:N);
%     iJ = J^(-1);
%     iJT = J.'^(-1);
%     
%     Mx = iJT*M.*iJ;
% taux = [Mx(1,1)*xdd(1)+Mx(1,2)*xdd(2); Mx(2,1)*xdd(1)+Mx(2,2)*xdd(2)];

== matlab function RRmanipulatorsim/MATLAB Function68 ==
  data: q input; taux output; qd input
function taux = Vx_Fx(q, qd)
    L = [1 1]; %Links long.
    m = [1 1]; %Links weight.
    
    M = [L(2)*m(2)*(L(2)+cos(q(2))*L(1))+m(1)*L(1)^2+L(1)*m(2)*(L(1)+cos(q(2))*L(2)) L(2)^2*m(2)+L(1)*m(2)*L(2)*cos(q(2));
        L(2)*m(2)*(L(2)+cos(q(2))*L(1)) L(2)^2*m(2)];
    V = [-2*m(2)*L(1)*L(2)*sin(q(2))*prod(qd)-m(2)*L(1)*L(2)*sin(q(2))*qd(2)^2;
        m(2)*L(1)*L(2)*sin(q(2))*qd(1)^2];
    G = [0;
        0];
    F = [sign(qd(1));
        sign(qd(2))];
    J = [-sin(sum(q))*L(2)-sin(q(1))*L(1) -sin(sum(q))*L(2);
        cos(sum(q))*L(2)+cos(q(1))*L(1) cos(sum(q))*L(2)];
    iJ = J^(-1);
    iJT = (J')^(-1);
    dJ = [-(sum(qd))*cos(sum(q))*L(2)-qd(1)*cos(q(1))*L(1) -(sum(qd))*cos(sum(q))*L(2);
        -(sum(qd))*sin(sum(q))*L(2)-qd(1)*sin(q(1))*L(1) -(sum(qd))*sin(sum(q))*L(2)];
    
    %dJqd = [dJ(1,1)*qd(1)+dJ(1,2)*qd(2); dJ(2,1)*qd(1)+dJ(2,2)*qd(2)];
    Vx = M*iJ*dJ;
    Vx = V - [Vx(1,1)*qd(1)+Vx(1,2)*qd(2); Vx(2,1)*qd(1)+Vx(2,2)*qd(2)];
    Vx = [iJT(1,1)*Vx(1)+iJT(1,2)*Vx(2); iJT(2,1)*Vx(1)+iJT(2,2)*Vx(2)];
    Gx = [iJT(1,1)*G(1)+iJT(1,2)*G(2); iJT(2,1)*G(1)+iJT(2,2)*G(2)];
    Fx = [iJT(1,1)*F(1)+iJT(1,2)*F(2); iJT(2,1)*F(1)+iJT(2,2)*F(2)];
taux = Vx + Gx + Fx;

% function taux = Vx_Fx(q, qd)
%     C = RRbot.coriolis(q', qd');
%     V = [C(1,1)*qd(1)+C(1,2)*qd(2); C(2,1)*qd(1)+C(2,2)*qd(2)]; %V = Cqd
%     F = -RRbot.friction(qd')';
%     J = RRbot.jacob0(q');
%     J = J(1:N,1:N);
%     iJ = J^(-1);
%     iJT = J.'^(-1);
%     dJ = [-(sum(qd))*cos(sum(q))*LT-qd(1)*cos(q(1))*L1 -(sum(qd))*cos(sum(q))*LT;
%         -(sum(qd))*sin(sum(q))*LT-qd(1)*sin(q(1))*L1 -(sum(qd))*sin(sum(q))*LT];
%     dJqd = [dJ(1,1)*qd(1)+dJ(1,2)*qd(2); dJ(2,1)*qd(1)+dJ(2,2)*qd(2)];
%     
%     Vx = M*iJ;
%     Vx = V - [Vx(1,1)*dJqd(1)+Vx(1,2)*dJqd(2); Vx(2,1)*dJqd(1)+Vx(2,2)*dJqd(2)];
%     Vx = [iJT(1,1)*Vx(1)+iJT(1,2)*Vx(2); iJT(2,1)*Vx(1)+iJT(2,2)*Vx(2)];
%     Fx = [iJT(1,1)*F(1)+iJT(1,2)*F(2); iJT(2,1)*F(1)+iJT(2,2)*F(2)];
% taux = Vx + Fx;

== matlab function RRmanipulatorsim/MATLAB Function69 ==
  data: q input; x output
function x = kine(q)
    L = [1 1]; %Links long.

x = [cos(sum(q))*L(2)+cos(q(1))*L(1); sin(sum(q))*L(2)+sin(q(1))*L(1)];

== matlab function RRmanipulatorsim/MATLAB Function70 ==
  data: q input; xd output; qd input
function xd = J(q, qd)
    L = [1 1]; %Links long.

    J = [-sin(sum(q))*L(2)-sin(q(1))*L(1) -sin(sum(q))*L(2);
        cos(sum(q))*L(2)+cos(q(1))*L(1) cos(sum(q))*L(2)];
xd = [J(1,1)*qd(1)+J(1,2)*qd(2); J(2,1)*qd(1)+J(2,2)*qd(2)];

== matlab function RRmanipulatorsim/MATLAB Function71 ==
  data: q input; tau output; taux input
function tau = JT(q, taux)    
    L = [1 1]; %Links long.

    J = [-sin(sum(q))*L(2)-sin(q(1))*L(1) -sin(sum(q))*L(2);
        cos(sum(q))*L(2)+cos(q(1))*L(1) cos(sum(q))*L(2)];
    JT = J';
tau = [JT(1,1)*taux(1)+JT(1,2)*taux(2); JT(2,1)*taux(1)+JT(2,2)*taux(2)];

% function tau = JT(q, taux)
%     J = RRbot.jacob0(q');
%     JT = J(1:N,1:N)';
% tau = [JT(1,1)*taux(1)+JT(1,2)*taux(2); JT(2,1)*taux(1)+JT(2,2)*taux(2)];

== matlab function RRmanipulatorsim/MATLAB Function72 ==
  data: x input; q output
function q = ikine(x)
    L = [1 1]; %Links long.
    
    C2 = (x(1)^2+x(2)^2-L(1)^2-L(2)^2)/(2*prod(L));
    S2 = sqrt(1-C2^2);
q = [atan2(x(2), x(1))-atan2(L(2)*S2, L(1)+L(2)*C2); atan2(S2, C2)];

== matlab function RRmanipulatorsim/MATLAB Function83 ==
  data: q input; taux output; xdd input
function taux = Mx(q, xdd)
    L = [1 1]; %Links long.
    m = [1 1]; %Links weight.
    
    M = [L(2)*m(2)*(L(2)+cos(q(2))*L(1))+m(1)*L(1)^2+L(1)*m(2)*(L(1)+cos(q(2))*L(2)) L(2)^2*m(2)+L(1)*m(2)*L(2)*cos(q(2));
        L(2)*m(2)*(L(2)+cos(q(2))*L(1)) L(2)^2*m(2)];
    J = [-sin(sum(q))*L(2)-sin(q(1))*L(1) -sin(sum(q))*L(2);
        cos(sum(q))*L(2)+cos(q(1))*L(1) cos(sum(q))*L(2)];
    iJ = J^(-1);
    iJT = (J.')^(-1);
    
    Mx = iJT*M*iJ;
taux = [Mx(1,1)*xdd(1)+Mx(1,2)*xdd(2); Mx(2,1)*xdd(1)+Mx(2,2)*xdd(2)];

% function taux = Mx(q, xdd)
%     M = RRbot.inertia(q');
%     J = RRbot.jacob0(q');
%     J = J(1:N,1:N);
%     iJ = J^(-1);
%     iJT = J.'^(-1);
%     
%     Mx = iJT*M.*iJ;
% taux = [Mx(1,1)*xdd(1)+Mx(1,2)*xdd(2); Mx(2,1)*xdd(1)+Mx(2,2)*xdd(2)];

== matlab function RRmanipulatorsim/MATLAB Function84 ==
  data: q input; taux output; qd input
function taux = Vx_Fx(q, qd)
    L = [1 1]; %Links long.
    m = [1 1]; %Links weight.
    
    M = [L(2)*m(2)*(L(2)+cos(q(2))*L(1))+m(1)*L(1)^2+L(1)*m(2)*(L(1)+cos(q(2))*L(2)) L(2)^2*m(2)+L(1)*m(2)*L(2)*cos(q(2));
        L(2)*m(2)*(L(2)+cos(q(2))*L(1)) L(2)^2*m(2)];
    V = [-2*m(2)*L(1)*L(2)*sin(q(2))*prod(qd)-m(2)*L(1)*L(2)*sin(q(2))*qd(2)^2;
        m(2)*L(1)*L(2)*sin(q(2))*qd(1)^2];
    G = [0;
        0];
    F = [sign(qd(1));
        sign(qd(2))];
    J = [-sin(sum(q))*L(2)-sin(q(1))*L(1) -sin(sum(q))*L(2);
        cos(sum(q))*L(2)+cos(q(1))*L(1) cos(sum(q))*L(2)];
    iJ = J^(-1);
    iJT = (J')^(-1);
    dJ = [-(sum(qd))*cos(sum(q))*L(2)-qd(1)*cos(q(1))*L(1) -(sum(qd))*cos(sum(q))*L(2);
        -(sum(qd))*sin(sum(q))*L(2)-qd(1)*sin(q(1))*L(1) -(sum(qd))*sin(sum(q))*L(2)];
    
    %dJqd = [dJ(1,1)*qd(1)+dJ(1,2)*qd(2); dJ(2,1)*qd(1)+dJ(2,2)*qd(2)];
    Vx = M*iJ*dJ;
    Vx = V - [Vx(1,1)*qd(1)+Vx(1,2)*qd(2); Vx(2,1)*qd(1)+Vx(2,2)*qd(2)];
    Vx = [iJT(1,1)*Vx(1)+iJT(1,2)*Vx(2); iJT(2,1)*Vx(1)+iJT(2,2)*Vx(2)];
    Gx = [iJT(1,1)*G(1)+iJT(1,2)*G(2); iJT(2,1)*G(1)+iJT(2,2)*G(2)];
    Fx = [iJT(1,1)*F(1)+iJT(1,2)*F(2); iJT(2,1)*F(1)+iJT(2,2)*F(2)];
taux = Vx + Gx + Fx;

% function taux = Vx_Fx(q, qd)
%     C = RRbot.coriolis(q', qd');
%     V = [C(1,1)*qd(1)+C(1,2)*qd(2); C(2,1)*qd(1)+C(2,2)*qd(2)]; %V = Cqd
%     F = -RRbot.friction(qd')';
%     J = RRbot.jacob0(q');
%     J = J(1:N,1:N);
%     iJ = J^(-1);
%     iJT = J.'^(-1);
%     dJ = [-(sum(qd))*cos(sum(q))*LT-qd(1)*cos(q(1))*L1 -(sum(qd))*cos(sum(q))*LT;
%         -(sum(qd))*sin(sum(q))*LT-qd(1)*sin(q(1))*L1 -(sum(qd))*sin(sum(q))*LT];
%     dJqd = [dJ(1,1)*qd(1)+dJ(1,2)*qd(2); dJ(2,1)*qd(1)+dJ(2,2)*qd(2)];
%     
%     Vx = M*iJ;
%     Vx = V - [Vx(1,1)*dJqd(1)+Vx(1,2)*dJqd(2); Vx(2,1)*dJqd(1)+Vx(2,2)*dJqd(2)];
%     Vx = [iJT(1,1)*Vx(1)+iJT(1,2)*Vx(2); iJT(2,1)*Vx(1)+iJT(2,2)*Vx(2)];
%     Fx = [iJT(1,1)*F(1)+iJT(1,2)*F(2); iJT(2,1)*F(1)+iJT(2,2)*F(2)];
% taux = Vx + Fx;

== matlab function RRmanipulatorsim/MATLAB Function85 ==
  data: q input; x output
function x = kine(q)
    L = [1 1]; %Links long.

x = [cos(sum(q))*L(2)+cos(q(1))*L(1); sin(sum(q))*L(2)+sin(q(1))*L(1)];

== matlab function RRmanipulatorsim/MATLAB Function86 ==
  data: q input; xd output; qd input
function xd = J(q, qd)
    L = [1 1]; %Links long.

    J = [-sin(sum(q))*L(2)-sin(q(1))*L(1) -sin(sum(q))*L(2);
        cos(sum(q))*L(2)+cos(q(1))*L(1) cos(sum(q))*L(2)];
xd = [J(1,1)*qd(1)+J(1,2)*qd(2); J(2,1)*qd(1)+J(2,2)*qd(2)];

== matlab function RRmanipulatorsim/MATLAB Function6 ==
  data: q input; x output
function x = kine(q)
    L = [1 1]; %Links long.

x = [cos(sum(q))*L(2)+cos(q(1))*L(1); sin(sum(q))*L(2)+sin(q(1))*L(1)];

== matlab function RRmanipulatorsim/MATLAB Function87 ==
  data: q input; tau output; taux input
function tau = JT(q, taux)    
    L = [1 1]; %Links long.

    J = [-sin(sum(q))*L(2)-sin(q(1))*L(1) -sin(sum(q))*L(2);
        cos(sum(q))*L(2)+cos(q(1))*L(1) cos(sum(q))*L(2)];
    JT = J';
tau = [JT(1,1)*taux(1)+JT(1,2)*taux(2); JT(2,1)*taux(1)+JT(2,2)*taux(2)];

% function tau = JT(q, taux)
%     J = RRbot.jacob0(q');
%     JT = J(1:N,1:N)';
% tau = [JT(1,1)*taux(1)+JT(1,2)*taux(2); JT(2,1)*taux(1)+JT(2,2)*taux(2)];

== matlab function RRmanipulatorsim/MATLAB Function88 ==
  data: x input; q output
function q = ikine(x)
    L = [1 1]; %Links long.
    
    C2 = (x(1)^2+x(2)^2-L(1)^2-L(2)^2)/(2*prod(L));
    S2 = sqrt(1-C2^2);
q = [atan2(x(2), x(1))-atan2(L(2)*S2, L(1)+L(2)*C2); atan2(S2, C2)];

== matlab function RRmanipulatorsim/MATLAB Function89 ==
  data: q input; taux output; xdd input
function taux = Mx(q, xdd)
    L = [1 1]; %Links long.
    m = [1 1]; %Links weight.
    
    M = [L(2)*m(2)*(L(2)+cos(q(2))*L(1))+m(1)*L(1)^2+L(1)*m(2)*(L(1)+cos(q(2))*L(2)) L(2)^2*m(2)+L(1)*m(2)*L(2)*cos(q(2));
        L(2)*m(2)*(L(2)+cos(q(2))*L(1)) L(2)^2*m(2)];
    J = [-sin(sum(q))*L(2)-sin(q(1))*L(1) -sin(sum(q))*L(2);
        cos(sum(q))*L(2)+cos(q(1))*L(1) cos(sum(q))*L(2)];
    iJ = J^(-1);
    iJT = (J.')^(-1);
    
    Mx = iJT*M*iJ;
taux = [Mx(1,1)*xdd(1)+Mx(1,2)*xdd(2); Mx(2,1)*xdd(1)+Mx(2,2)*xdd(2)];

% function taux = Mx(q, xdd)
%     M = RRbot.inertia(q');
%     J = RRbot.jacob0(q');
%     J = J(1:N,1:N);
%     iJ = J^(-1);
%     iJT = J.'^(-1);
%     
%     Mx = iJT*M.*iJ;
% taux = [Mx(1,1)*xdd(1)+Mx(1,2)*xdd(2); Mx(2,1)*xdd(1)+Mx(2,2)*xdd(2)];

== matlab function RRmanipulatorsim/MATLAB Function90 ==
  data: q input; taux output; qd input
function taux = Vx_Fx(q, qd)
    L = [1 1]; %Links long.
    m = [1 1]; %Links weight.
    
    M = [L(2)*m(2)*(L(2)+cos(q(2))*L(1))+m(1)*L(1)^2+L(1)*m(2)*(L(1)+cos(q(2))*L(2)) L(2)^2*m(2)+L(1)*m(2)*L(2)*cos(q(2));
        L(2)*m(2)*(L(2)+cos(q(2))*L(1)) L(2)^2*m(2)];
    V = [-2*m(2)*L(1)*L(2)*sin(q(2))*prod(qd)-m(2)*L(1)*L(2)*sin(q(2))*qd(2)^2;
        m(2)*L(1)*L(2)*sin(q(2))*qd(1)^2];
    G = [0;
        0];
    F = [sign(qd(1));
        sign(qd(2))];
    J = [-sin(sum(q))*L(2)-sin(q(1))*L(1) -sin(sum(q))*L(2);
        cos(sum(q))*L(2)+cos(q(1))*L(1) cos(sum(q))*L(2)];
    iJ = J^(-1);
    iJT = (J')^(-1);
    dJ = [-(sum(qd))*cos(sum(q))*L(2)-qd(1)*cos(q(1))*L(1) -(sum(qd))*cos(sum(q))*L(2);
        -(sum(qd))*sin(sum(q))*L(2)-qd(1)*sin(q(1))*L(1) -(sum(qd))*sin(sum(q))*L(2)];
    
    %dJqd = [dJ(1,1)*qd(1)+dJ(1,2)*qd(2); dJ(2,1)*qd(1)+dJ(2,2)*qd(2)];
    Vx = M*iJ*dJ;
    Vx = V - [Vx(1,1)*qd(1)+Vx(1,2)*qd(2); Vx(2,1)*qd(1)+Vx(2,2)*qd(2)];
    Vx = [iJT(1,1)*Vx(1)+iJT(1,2)*Vx(2); iJT(2,1)*Vx(1)+iJT(2,2)*Vx(2)];
    Gx = [iJT(1,1)*G(1)+iJT(1,2)*G(2); iJT(2,1)*G(1)+iJT(2,2)*G(2)];
    Fx = [iJT(1,1)*F(1)+iJT(1,2)*F(2); iJT(2,1)*F(1)+iJT(2,2)*F(2)];
taux = Vx + Gx + Fx;

% function taux = Vx_Fx(q, qd)
%     C = RRbot.coriolis(q', qd');
%     V = [C(1,1)*qd(1)+C(1,2)*qd(2); C(2,1)*qd(1)+C(2,2)*qd(2)]; %V = Cqd
%     F = -RRbot.friction(qd')';
%     J = RRbot.jacob0(q');
%     J = J(1:N,1:N);
%     iJ = J^(-1);
%     iJT = J.'^(-1);
%     dJ = [-(sum(qd))*cos(sum(q))*LT-qd(1)*cos(q(1))*L1 -(sum(qd))*cos(sum(q))*LT;
%         -(sum(qd))*sin(sum(q))*LT-qd(1)*sin(q(1))*L1 -(sum(qd))*sin(sum(q))*LT];
%     dJqd = [dJ(1,1)*qd(1)+dJ(1,2)*qd(2); dJ(2,1)*qd(1)+dJ(2,2)*qd(2)];
%     
%     Vx = M*iJ;
%     Vx = V - [Vx(1,1)*dJqd(1)+Vx(1,2)*dJqd(2); Vx(2,1)*dJqd(1)+Vx(2,2)*dJqd(2)];
%     Vx = [iJT(1,1)*Vx(1)+iJT(1,2)*Vx(2); iJT(2,1)*Vx(1)+iJT(2,2)*Vx(2)];
%     Fx = [iJT(1,1)*F(1)+iJT(1,2)*F(2); iJT(2,1)*F(1)+iJT(2,2)*F(2)];
% taux = Vx + Fx;

== matlab function RRmanipulatorsim/MATLAB Function91 ==
  data: q input; x output
function x = kine(q)
    L = [1 1]; %Links long.

x = [cos(sum(q))*L(2)+cos(q(1))*L(1); sin(sum(q))*L(2)+sin(q(1))*L(1)];

== matlab function RRmanipulatorsim/MATLAB Function92 ==
  data: q input; xd output; qd input
function xd = J(q, qd)
    L = [1 1]; %Links long.

    J = [-sin(sum(q))*L(2)-sin(q(1))*L(1) -sin(sum(q))*L(2);
        cos(sum(q))*L(2)+cos(q(1))*L(1) cos(sum(q))*L(2)];
xd = [J(1,1)*qd(1)+J(1,2)*qd(2); J(2,1)*qd(1)+J(2,2)*qd(2)];

== matlab function RRmanipulatorsim/MATLAB Function93 ==
  data: q input; tau output; taux input
function tau = JT(q, taux)    
    L = [1 1]; %Links long.

    J = [-sin(sum(q))*L(2)-sin(q(1))*L(1) -sin(sum(q))*L(2);
        cos(sum(q))*L(2)+cos(q(1))*L(1) cos(sum(q))*L(2)];
    JT = J';
tau = [JT(1,1)*taux(1)+JT(1,2)*taux(2); JT(2,1)*taux(1)+JT(2,2)*taux(2)];

% function tau = JT(q, taux)
%     J = RRbot.jacob0(q');
%     JT = J(1:N,1:N)';
% tau = [JT(1,1)*taux(1)+JT(1,2)*taux(2); JT(2,1)*taux(1)+JT(2,2)*taux(2)];

== matlab function RRmanipulatorsim/MATLAB Function94 ==
  data: x input; q output
function q = ikine(x)
    L = [1 1]; %Links long.
    
    C2 = (x(1)^2+x(2)^2-L(1)^2-L(2)^2)/(2*prod(L));
    S2 = sqrt(1-C2^2);
q = [atan2(x(2), x(1))-atan2(L(2)*S2, L(1)+L(2)*C2); atan2(S2, C2)];

== matlab function RRmanipulatorsim/MATLAB Function100 ==
  data: x input; q output
function q = ikine(x)
    L = [1 1]; %Links long.
    
    C2 = (x(1)^2+x(2)^2-L(1)^2-L(2)^2)/(2*prod(L));
    S2 = sqrt(1-C2^2);
q = [atan2(x(2), x(1))-atan2(L(2)*S2, L(1)+L(2)*C2); atan2(S2, C2)];

== matlab function RRmanipulatorsim/MATLAB Function7 ==
  data: q input; xd output; qd input
function xd = J(q, qd)
    L = [1 1]; %Links long.

    J = [-sin(sum(q))*L(2)-sin(q(1))*L(1) -sin(sum(q))*L(2);
        cos(sum(q))*L(2)+cos(q(1))*L(1) cos(sum(q))*L(2)];
xd = [J(1,1)*qd(1)+J(1,2)*qd(2); J(2,1)*qd(1)+J(2,2)*qd(2)];

== matlab function RRmanipulatorsim/MATLAB Function101 ==
  data: q input; taux output; xdd input
function taux = Mx(q, xdd)
    L = [1 1]; %Links long.
    m = [1 1]; %Links weight.
    
    M = [L(2)*m(2)*(L(2)+cos(q(2))*L(1))+m(1)*L(1)^2+L(1)*m(2)*(L(1)+cos(q(2))*L(2)) L(2)^2*m(2)+L(1)*m(2)*L(2)*cos(q(2));
        L(2)*m(2)*(L(2)+cos(q(2))*L(1)) L(2)^2*m(2)];
    J = [-sin(sum(q))*L(2)-sin(q(1))*L(1) -sin(sum(q))*L(2);
        cos(sum(q))*L(2)+cos(q(1))*L(1) cos(sum(q))*L(2)];
    iJ = J^(-1);
    iJT = (J.')^(-1);
    
    Mx = iJT*M*iJ;
taux = [Mx(1,1)*xdd(1)+Mx(1,2)*xdd(2); Mx(2,1)*xdd(1)+Mx(2,2)*xdd(2)];

% function taux = Mx(q, xdd)
%     M = RRbot.inertia(q');
%     J = RRbot.jacob0(q');
%     J = J(1:N,1:N);
%     iJ = J^(-1);
%     iJT = J.'^(-1);
%     
%     Mx = iJT*M.*iJ;
% taux = [Mx(1,1)*xdd(1)+Mx(1,2)*xdd(2); Mx(2,1)*xdd(1)+Mx(2,2)*xdd(2)];

== matlab function RRmanipulatorsim/MATLAB Function102 ==
  data: q input; taux output; qd input
function taux = Vx_Fx(q, qd)
    L = [1 1]; %Links long.
    m = [1 1]; %Links weight.
    
    M = [L(2)*m(2)*(L(2)+cos(q(2))*L(1))+m(1)*L(1)^2+L(1)*m(2)*(L(1)+cos(q(2))*L(2)) L(2)^2*m(2)+L(1)*m(2)*L(2)*cos(q(2));
        L(2)*m(2)*(L(2)+cos(q(2))*L(1)) L(2)^2*m(2)];
    V = [-2*m(2)*L(1)*L(2)*sin(q(2))*prod(qd)-m(2)*L(1)*L(2)*sin(q(2))*qd(2)^2;
        m(2)*L(1)*L(2)*sin(q(2))*qd(1)^2];
    G = [0;
        0];
    F = [sign(qd(1));
        sign(qd(2))];
    J = [-sin(sum(q))*L(2)-sin(q(1))*L(1) -sin(sum(q))*L(2);
        cos(sum(q))*L(2)+cos(q(1))*L(1) cos(sum(q))*L(2)];
    iJ = J^(-1);
    iJT = (J')^(-1);
    dJ = [-(sum(qd))*cos(sum(q))*L(2)-qd(1)*cos(q(1))*L(1) -(sum(qd))*cos(sum(q))*L(2);
        -(sum(qd))*sin(sum(q))*L(2)-qd(1)*sin(q(1))*L(1) -(sum(qd))*sin(sum(q))*L(2)];
    
    %dJqd = [dJ(1,1)*qd(1)+dJ(1,2)*qd(2); dJ(2,1)*qd(1)+dJ(2,2)*qd(2)];
    Vx = M*iJ*dJ;
    Vx = V - [Vx(1,1)*qd(1)+Vx(1,2)*qd(2); Vx(2,1)*qd(1)+Vx(2,2)*qd(2)];
    Vx = [iJT(1,1)*Vx(1)+iJT(1,2)*Vx(2); iJT(2,1)*Vx(1)+iJT(2,2)*Vx(2)];
    Gx = [iJT(1,1)*G(1)+iJT(1,2)*G(2); iJT(2,1)*G(1)+iJT(2,2)*G(2)];
    Fx = [iJT(1,1)*F(1)+iJT(1,2)*F(2); iJT(2,1)*F(1)+iJT(2,2)*F(2)];
taux = Vx + Gx + Fx;

% function taux = Vx_Fx(q, qd)
%     C = RRbot.coriolis(q', qd');
%     V = [C(1,1)*qd(1)+C(1,2)*qd(2); C(2,1)*qd(1)+C(2,2)*qd(2)]; %V = Cqd
%     F = -RRbot.friction(qd')';
%     J = RRbot.jacob0(q');
%     J = J(1:N,1:N);
%     iJ = J^(-1);
%     iJT = J.'^(-1);
%     dJ = [-(sum(qd))*cos(sum(q))*LT-qd(1)*cos(q(1))*L1 -(sum(qd))*cos(sum(q))*LT;
%         -(sum(qd))*sin(sum(q))*LT-qd(1)*sin(q(1))*L1 -(sum(qd))*sin(sum(q))*LT];
%     dJqd = [dJ(1,1)*qd(1)+dJ(1,2)*qd(2); dJ(2,1)*qd(1)+dJ(2,2)*qd(2)];
%     
%     Vx = M*iJ;
%     Vx = V - [Vx(1,1)*dJqd(1)+Vx(1,2)*dJqd(2); Vx(2,1)*dJqd(1)+Vx(2,2)*dJqd(2)];
%     Vx = [iJT(1,1)*Vx(1)+iJT(1,2)*Vx(2); iJT(2,1)*Vx(1)+iJT(2,2)*Vx(2)];
%     Fx = [iJT(1,1)*F(1)+iJT(1,2)*F(2); iJT(2,1)*F(1)+iJT(2,2)*F(2)];
% taux = Vx + Fx;
